simulink model "pneumatics"  (R2025a)
settings: Solver=ode8  StartTime=0.0  StopTime=10  FixedStep=0.01  RelTol=1e-3
model workspace (MAT data in the model file):
  BP_MAX_SERVICE_REDUCTION = Simulink.Parameter
  BP_MAX_SERVICE_REDUCTION.Value = 25
  BP_MAX_SERVICE_REDUCTION.Complexity = 'real'
  BP_MAX_SERVICE_REDUCTION.Dimensions = [1 1]
  BP_MAX_SERVICE_REDUCTION.DataType = 'auto'
  BP_MAX_SERVICE_REDUCTION.DocUnits = 'psig'
  BP_NOMINAL_PRESSURE = Simulink.Parameter
  BP_NOMINAL_PRESSURE.Value = 104.69
  BP_NOMINAL_PRESSURE.Complexity = 'real'
  BP_NOMINAL_PRESSURE.Dimensions = [1 1]
  BP_NOMINAL_PRESSURE.DataType = 'auto'
  BP_NOMINAL_PRESSURE.DocUnits = 'psia'
  MAIN_RES_NOMINAL_PRESSURE = Simulink.Parameter
  MAIN_RES_NOMINAL_PRESSURE.Value = 154.69
  MAIN_RES_NOMINAL_PRESSURE.Complexity = 'real'
  MAIN_RES_NOMINAL_PRESSURE.Dimensions = [1 1]
  MAIN_RES_NOMINAL_PRESSURE.DataType = 'auto'
  MAIN_RES_NOMINAL_PRESSURE.DocUnits = 'psia'
  RESERVOIR_TEMPERATURE = Simulink.Parameter
  RESERVOIR_TEMPERATURE.Value = 75
  RESERVOIR_TEMPERATURE.Complexity = 'real'
  RESERVOIR_TEMPERATURE.Dimensions = [1 1]
  RESERVOIR_TEMPERATURE.DataType = 'auto'
  RESERVOIR_TEMPERATURE.DocUnits = '°F'
  RESERVOIR_VOLUME = Simulink.Parameter
  RESERVOIR_VOLUME.Value = 10
  RESERVOIR_VOLUME.Complexity = 'real'
  RESERVOIR_VOLUME.Dimensions = [1 1]
  RESERVOIR_VOLUME.DataType = 'auto'
  RESERVOIR_VOLUME.DocUnits = 'gal'
  TRANSDUCER_ADC_OUTPUT_RANGE = Simulink.Parameter
  TRANSDUCER_ADC_OUTPUT_RANGE.Value = 1019
  TRANSDUCER_ADC_OUTPUT_RANGE.Complexity = 'real'
  TRANSDUCER_ADC_OUTPUT_RANGE.Dimensions = [1 1]
  TRANSDUCER_ADC_OUTPUT_RANGE.DataType = 'auto'
  TRANSDUCER_ADC_OUTPUT_RANGE.DocUnits = 'bit'
  TRANSDUCER_OUTPUT_HIGH = Simulink.Parameter
  TRANSDUCER_OUTPUT_HIGH.Value = 4.5
  TRANSDUCER_OUTPUT_HIGH.Complexity = 'real'
  TRANSDUCER_OUTPUT_HIGH.Dimensions = [1 1]
  TRANSDUCER_OUTPUT_HIGH.DataType = 'auto'
  TRANSDUCER_OUTPUT_LOW = Simulink.Parameter
  TRANSDUCER_OUTPUT_LOW.Value = 0.5
  TRANSDUCER_OUTPUT_LOW.Complexity = 'real'
  TRANSDUCER_OUTPUT_LOW.Dimensions = [1 1]
  TRANSDUCER_OUTPUT_LOW.DataType = 'auto'
  TRANSDUCER_OUTPUT_RANGE = Simulink.Parameter
  TRANSDUCER_OUTPUT_RANGE.Value = 4
  TRANSDUCER_OUTPUT_RANGE.Complexity = 'real'
  TRANSDUCER_OUTPUT_RANGE.Dimensions = [1 1]
  TRANSDUCER_OUTPUT_RANGE.DataType = 'auto'
  TRANSDUCER_OUTPUT_RANGE.DocUnits = 'V'
  TRANSDUCER_PRESSURE_RANGE = Simulink.Parameter
  TRANSDUCER_PRESSURE_RANGE.Value = 150
  TRANSDUCER_PRESSURE_RANGE.Complexity = 'real'
  TRANSDUCER_PRESSURE_RANGE.Dimensions = [1 1]
  TRANSDUCER_PRESSURE_RANGE.DataType = 'auto'
  TRANSDUCER_PRESSURE_RANGE.DocUnits = 'psig'
values from neighbouring files (symbols this model uses):
  max_bc_pressure = 50.0    [pneumatics.sldd]
settings Model: DataDictionary=pneumatics.sldd  ExtModeTrigDuration=100  Creator=adam  LastModifiedBy=adam
settings SolverCC: MaxConsecutiveMinStep=3
settings DataIOCC: SaveFormat=Array  SaveOutput=off
settings OptimizationCC: DefaultParameterBehavior=Inlined  InlineInvariantSignals=on  EnhancedBackFolding=on  PassReuseOutputArgsThreshold=0.0  OptimizeBlockOrder=speed  DifferentSizesBufferReuse=on  OptimizationCustomize=off
settings DebuggingCC: ParameterTunabilityLossMsg=error
settings HardwareCC: TargetBitPerLong=64.0  TargetBitPerPointer=64.0  TargetBitPerSizeT=64.0  TargetBitPerPtrDiffT=64.0  TargetLongLongMode=on  TargetIntDivRoundTo=Zero  TargetEndianess=LittleEndian  TargetWordSize=64.0  TargetHWDeviceType=MATLAB Host  ProdEqTarget=off
settings SFSimCC: MATLABDynamicMemAlloc=off
settings RTWCC: PackageGeneratedCodeAndArtifacts=on  RetainRTWFile=on  GPUComputeCapability=3.5
settings CodeAppCC: ForceParamTrailComments=on  MaxIdLength=95.0  OperatorAnnotations=on
settings SimscapeCC: SimscapeLogOpenViewer=on  SimscapeLogLimitData=off  SimscapeCacheCompileArtifacts=off

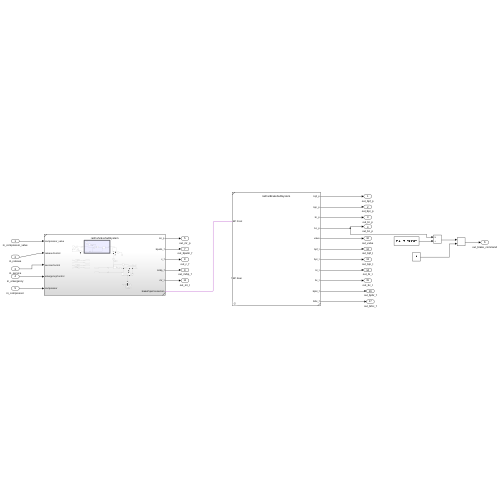
[thumbnail: Simulink's stored preview of the top-level diagram]
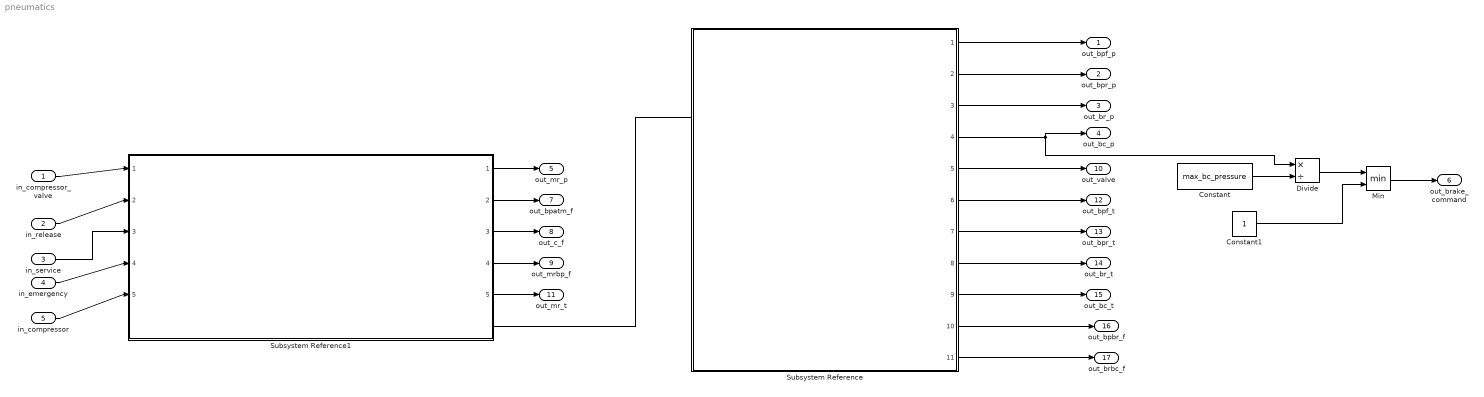
== system pneumatics ==
  in_compressor_valve : Inport
  in_release : Inport  Port=2
  in_service : Inport  Port=3
  in_emergency : Inport  Port=4
  in_compressor : Inport  Port=5
  Constant : Constant  Value=max_bc_pressure
  Constant1 : Constant
  Divide : Product  Inputs=*/
  Min : MinMax  Inputs=2
  Subsystem Reference : Subsystem  ReferencedSubsystem=railCarBrakeSubSystem  reservoir_temperature=RESERVOIR_TEMPERATURE degF  p_init=BP_NOMINAL_PRESSURE psi  r_volume=10 gal  bc_volume=4 gal  bc_pressure=14.69 psi  length=50 ft  area=1.23 in^2  Dh=1.25 in
  Subsystem Reference1 : Subsystem  ReferencedSubsystem=railCarValveSubSystem
  out_bpf_p : Outport
  out_bpr_p : Outport  Port=2
  out_br_p : Outport  Port=3
  out_bc_p : Outport  Port=4
  out_mr_p : Outport  Port=5
  out_brake_command : Outport  Port=6
  out_bpatm_f : Outport  Port=7
  out_c_f : Outport  Port=8
  out_mrbp_f : Outport  Port=9
  out_valve : Outport  Port=10
  out_mr_t : Outport  Port=11
  out_bpf_t : Outport  Port=12
  out_bpr_t : Outport  Port=13
  out_br_t : Outport  Port=14
  out_bc_t : Outport  Port=15
  out_bpbr_f : Outport  Port=16
  out_brbc_f : Outport  Port=17
  wires:
  Subsystem Reference1/1 -> out_mr_p/1
  Subsystem Reference/1 -> out_bpf_p/1
  Subsystem Reference/2 -> out_bpr_p/1
  Subsystem Reference/3 -> out_br_p/1
  Subsystem Reference/4 -> out_bc_p/1, Divide/1
  in_compressor_valve/1 -> Subsystem Reference1/1
  in_release/1 -> Subsystem Reference1/2
  in_service/1 -> Subsystem Reference1/3
  in_emergency/1 -> Subsystem Reference1/4
  Constant/1 -> Divide/2
  Min/1 -> out_brake_command/1
  Divide/1 -> Min/1
  Constant1/1 -> Min/2
  Subsystem Reference1/2 -> out_bpatm_f/1
  Subsystem Reference1/4 -> out_mrbp_f/1
  Subsystem Reference1/3 -> out_c_f/1
  Subsystem Reference/5 -> out_valve/1
  Subsystem Reference1/5 -> out_mr_t/1
  Subsystem Reference/6 -> out_bpf_t/1
  Subsystem Reference/7 -> out_bpr_t/1
  Subsystem Reference/8 -> out_br_t/1
  Subsystem Reference/9 -> out_bc_t/1
  Subsystem Reference/11 -> out_brbc_f/1
  Subsystem Reference/10 -> out_bpbr_f/1
  in_compressor/1 -> Subsystem Reference1/5
  connections:
  Subsystem Reference1/RConn1 -- Subsystem Reference/LConn1
